simulink model "UGRP_Drone_Modeling4_with_motor_dynamics_v2_with_state_space"  (R2021b)
settings: Solver=FixedStepAuto  StartTime=0.0  StopTime=27  FixedStep=1/600
undefined symbols (not defined in the file or in its folder): sigbuilder_block
libraries: simulink x1, sim3dlib x1, uavsim3dlib x1
settings Model: Creator=user  LastModifiedBy=user
settings SolverCC: MaxConsecutiveMinStep=5  ShapePreserveControl=EnableAll  ZeroCrossAlgorithm=Adaptive
settings DebuggingCC: MaskedZcDiagnostic=none  IgnoredZcDiagnostic=none
settings SFSimCC: SimHardwareAcceleration=native  SimTargetLang=C++

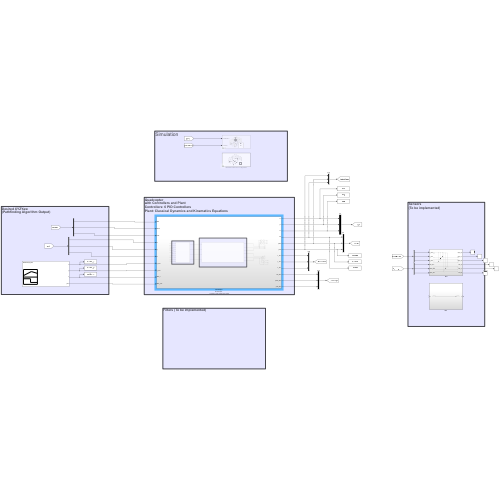
[thumbnail: Simulink's stored preview of the top-level diagram]
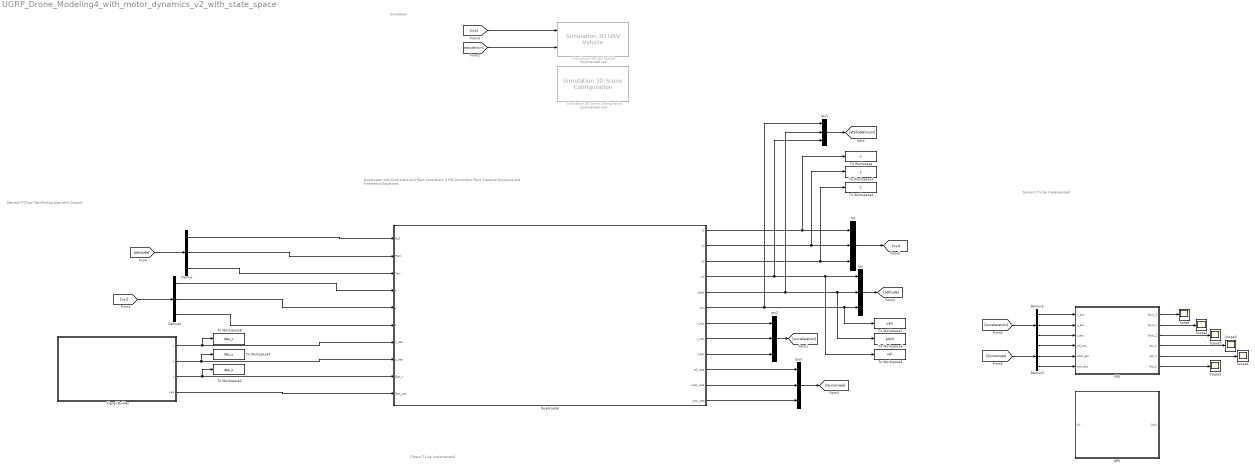
== system UGRP_Drone_Modeling4_with_motor_dynamics_v2_with_state_space ==
  note: Filters (To be implemented)
  note: Sensors
      | (To be implemented)
  note: Desired XYZYaw
      | (Pathfinding Algorithm Output)
  note: Quadcopter
      | with Controllers and Plant
      | Controllers: 6 PID Controllers
      | Plant: Classical Dynamics and Kinematics Equations
  note: Simulation
  Demux{,1..3} (4 alike) : Demux  Outputs=3
  GPS : Subsystem
  IMU : Subsystem
  Quadcopter : Subsystem  Description=Quadcopter including controllers and plant
      settings: AttributesFormatString=|
      | Quadcopter
      | - Controller and Quadcopter Plant
  Scope{,1..5} (6 alike) : Scope
  Signal Builder : Subsystem  Tag=STV Subsys  LoadFcn=sigbuilder_block('load',[10.5 -27.75 821.25 385.5 ]);  StartFcn=sigbuilder_block('start');  StopFcn=sigbuilder_block('stop');  ClipboardFcn=sigbuilder_block('clipboard');  mask(Sigbuilder block){tuvar=[0:10]}
      mask help: Simulink:masks:SigbuilderBlock_MD
      mask init:
      | if ~strcmp(get_param(bdroot(gcbh),'SimulationStatus'),'stopped') tuvar = sigbuilder_block('maskInit'); end
      settings: CopyFcn=sigbuilder_block('copy');  DeleteFcn=sigbuilder_block('delete');  ModelCloseFcn=sigbuilder_block('modelClose');  PreSaveFcn=sigbuilder_block('preSave');  PauseFcn=sigbuilder_block('pause');  ContinueFcn=sigbuilder_block('continue');  NameChangeFcn=sigbuilder_block('namechange');  OpenFcn=sigbuilder_block('open',[9 69.75 821.25 385.5 ]);  CloseFcn=sigbuilder_block('close');
      mask Display: plot(0, 0, 100, 100,[2, 2, 32, 32, 2], [68, 8, 8, 68, 68],[32, 2], [38, 38], [32, 19, 2],[53, 60, 44], [32, 17, 17, 2],[16, 16, 31, 31]);txt = getActiveGroup(gcbh);text(2, 100, txt,'verticalAlignment', 'top');
  Simulation 3D Scene Configuration : sim3dlib/Simulation 3D Scene Configuration  Priority=0  Commented=on  ProjectFormat_internal=Default Scenes  ProjectFormat=Default Scenes  SceneDesc=US city block  ProjectName=C:\Program Files\MATLAB\R2021b\toolbox\shared\sim3d_projects\automotive_project\UE4\WindowsNoEditor\VehicleSimulation.exe  ScenePath=/Game/Maps/USCityBlock  vehTagList={'Scene Origin';'SimulinkVehicle1'}  vehTag=SimulinkVehicle1  OpVisEn=off  Ts=1/60  EnableWindow=on  EnableWeather=off  SunAltitude=40.0  SunAzimuth=90  clouds=10  wind=1  fog=0  rain=0  sensorTag=MainCamera1  sensorId=1  sensorName=MainCamera1  mountLoc=Origin  offsetFlag=off  tmountOffset=[0, 0, 0]  rmountOffset=[0, 0, 0]  HorizontalResolution=1280  VerticalResolution=720  HorizontalFOV=60  mountPoint=[0 0 0]  mountOrientation=[0 0 0]  aMode=4  ID=1
      settings: SourceProductBaseCode=AE,DR,UV,VE
  Simulation 3D UAV Vehicle : uavsim3dlib/Simulation 3D UAV Vehicle  Priority=-1  Commented=on  Mesh=Quadrotor  MeshPath=/MathWorksUAVContent/UAVs/HexaRotorUAV/HexaRotor.HexaRotor  Color=Black  ActorName=SimulinkVehicle1  InitialTranslation=[0 0 0]  InitialRotation=[0 0 0]  SampleTime=-1  ActorType=SimulinkVehicle  ID=1  aMode=4  ActorTag=SimulinkVehicle1
      settings: SourceProductBaseCode=UV
  To Workspace : ToWorkspace  VariableName=x  SaveFormat=Timeseries  SampleTime=-1
  To Workspace2 : ToWorkspace  VariableName=des_z  SaveFormat=Timeseries  SampleTime=-1
  To Workspace3 : ToWorkspace  VariableName=y  SaveFormat=Timeseries  SampleTime=-1
  To Workspace4 : ToWorkspace  VariableName=z  SaveFormat=Timeseries  SampleTime=-1
  To Workspace5 : ToWorkspace  VariableName=roll  SaveFormat=Timeseries  SampleTime=-1
  To Workspace6 : ToWorkspace  VariableName=pitch  SaveFormat=Timeseries  SampleTime=-1
  To Workspace7 : ToWorkspace  VariableName=yaw  SaveFormat=Timeseries  SampleTime=-1
  To Workspace8 : ToWorkspace  VariableName=des_x  SaveFormat=Timeseries  SampleTime=-1
  To Workspace9 : ToWorkspace  VariableName=des_y  SaveFormat=Timeseries  SampleTime=-1
  rpy{,1..3} (4 alike) : Mux  Inputs=3
  xyz : Mux  Inputs=3
  wires:
  Signal Builder/3(z) -> Quadcopter/9(Des_z), To Workspace2/1
  xyz/1 -> [xyz]
  rpy/1 -> [attitude]
  [xyz] -> Demux2/1
  [attitude] -> Demux/1
  Demux2/1 -> Quadcopter/4(x)
  Demux2/2 -> Quadcopter/5(y)
  Demux2/3 -> Quadcopter/6(z)
  Signal Builder/4(yaw) -> Quadcopter/10(Des_yaw)
  [xyz] -> Simulation 3D UAV Vehicle/1
  [attitudeforsim] -> Simulation 3D UAV Vehicle/2
  Signal Builder/1(x) -> Quadcopter/7(x_des), To Workspace8/1
  Signal Builder/2(y) -> Quadcopter/8(y_des), To Workspace9/1
  Quadcopter/1(x1) -> xyz/1, To Workspace/1
  Quadcopter/3(z1) -> To Workspace4/1, xyz/3
  Quadcopter/2(y1) -> To Workspace3/1, xyz/2
  Demux/1 -> Quadcopter/1(Roll)
  Demux/2 -> Quadcopter/2(Pitch)
  Demux/3 -> Quadcopter/3(Yaw)
  rpy1/1 -> [attitudeforsim]
  Quadcopter/4(roll) -> rpy1/3, To Workspace5/1, rpy/1
  Quadcopter/5(pitch) -> rpy1/2, To Workspace6/1, rpy/2
  Quadcopter/6(yaw) -> rpy1/1, To Workspace7/1, rpy/3
  Quadcopter/7(x_acc) -> rpy2/1
  Quadcopter/8(y_acc) -> rpy2/2
  Quadcopter/9(z_acc) -> rpy2/3
  Quadcopter/10(roll_rate) -> rpy3/1
  Quadcopter/11(pitch_rate) -> rpy3/2
  Quadcopter/12(yaw_rate) -> rpy3/3
  rpy2/1 -> [Acceleration]
  rpy3/1 -> [Gyroscope]
  [Acceleration] -> Demux1/1
  [Gyroscope] -> Demux3/1
  Demux1/1 -> IMU/1(x_acc)
  Demux1/2 -> IMU/2(y_acc)
  Demux1/3 -> IMU/3(z_acc)
  Demux3/1 -> IMU/4(roll_acc)
  Demux3/2 -> IMU/5(pitch_acc)
  Demux3/3 -> IMU/6(yaw_acc)
  IMU/1(Gyro_X) -> Scope/1
  IMU/2(Gyro_Y) -> Scope1/1
  IMU/3(Gyro_Z) -> Scope2/1
  IMU/4(Acc_X) -> Scope3/1
  IMU/5(Acc_Y) -> Scope4/1
  IMU/6(Acc_Z) -> Scope5/1

== system UGRP_Drone_Modeling4_with_motor_dynamics_v2_with_state_space/GPS ==
  In1 : Inport
  Out1 : Outport
  wires:
  In1/1 -> Out1/1

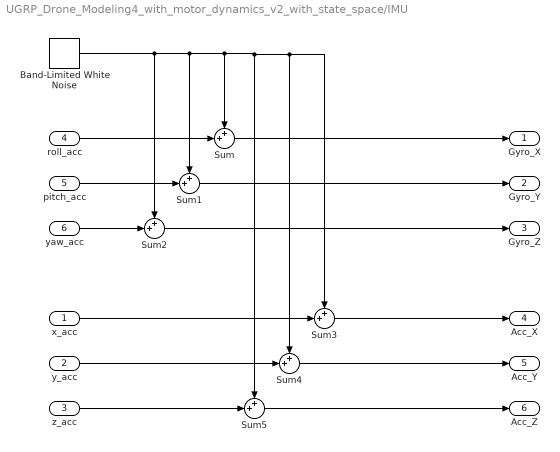
== system UGRP_Drone_Modeling4_with_motor_dynamics_v2_with_state_space/IMU ==
  x_acc : Inport
  y_acc : Inport  Port=2
  z_acc : Inport  Port=3
  roll_acc : Inport  Port=4
  pitch_acc : Inport  Port=5
  yaw_acc : Inport  Port=6
  Band-Limited White Noise : simulink/Sources/Band-Limited White Noise  Cov=[0.5]  Ts=0.1  seed=[23341]
  Sum{,1..5} (6 alike) : Sum  Inputs=++|
  Gyro_X : Outport
  Gyro_Y : Outport  Port=2
  Gyro_Z : Outport  Port=3
  Acc_X : Outport  Port=4
  Acc_Y : Outport  Port=5
  Acc_Z : Outport  Port=6
  wires:
  yaw_acc/1 -> Sum2/2
  pitch_acc/1 -> Sum1/2
  roll_acc/1 -> Sum/2
  Band-Limited White Noise/1 -> Sum3/1, Sum4/1, Sum5/1, Sum/1, Sum1/1, Sum2/1
  x_acc/1 -> Sum3/2
  y_acc/1 -> Sum4/2
  z_acc/1 -> Sum5/2
  Sum/1 -> Gyro_X/1
  Sum1/1 -> Gyro_Y/1
  Sum2/1 -> Gyro_Z/1
  Sum3/1 -> Acc_X/1
  Sum4/1 -> Acc_Y/1
  Sum5/1 -> Acc_Z/1

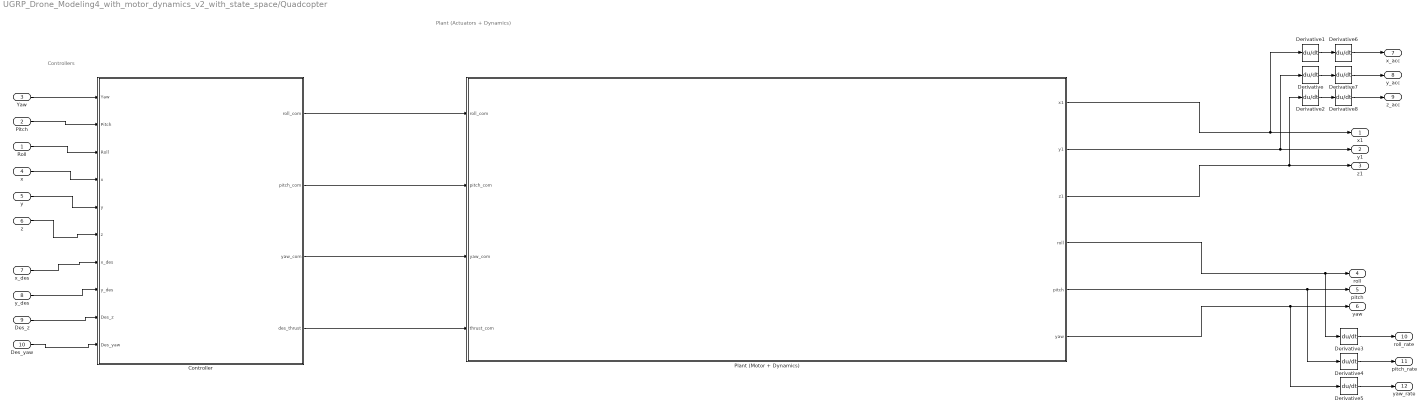
== system UGRP_Drone_Modeling4_with_motor_dynamics_v2_with_state_space/Quadcopter ==
  note: Plant (Actuators + Dynamics)
  note: Controllers
  Roll : Inport
  Pitch : Inport  Port=2
  Yaw : Inport  Port=3
  x : Inport  Port=4
  y : Inport  Port=5
  z : Inport  Port=6
  x_des : Inport  Port=7
  y_des : Inport  Port=8
  Des_z : Inport  Port=9
  Des_yaw : Inport  Port=10
  Controller : Subsystem
  Derivative{,1..8} (9 alike) : Derivative
  Plant (Motor + Dynamics) : Subsystem
  x1 : Outport
  y1 : Outport  Port=2
  z1 : Outport  Port=3
  roll : Outport  Port=4
  pitch : Outport  Port=5
  yaw : Outport  Port=6
  x_acc : Outport  Port=7
  y_acc : Outport  Port=8
  z_acc : Outport  Port=9
  roll_rate : Outport  Port=10
  pitch_rate : Outport  Port=11
  yaw_rate : Outport  Port=12
  wires:
  x_des/1 -> Controller/7(x_des)
  Controller/1(roll_com) -> Plant (Motor + Dynamics)/1(roll_com)
  Controller/2(pitch_com) -> Plant (Motor + Dynamics)/2(pitch_com)
  Des_yaw/1 -> Controller/10(Des_yaw)
  Controller/4(des_thrust) -> Plant (Motor + Dynamics)/4(thrust_com)
  Controller/3(yaw_com) -> Plant (Motor + Dynamics)/3(yaw_com)
  y/1 -> Controller/5(y)
  Des_z/1 -> Controller/9(Des_z)
  x/1 -> Controller/4(x)
  Roll/1 -> Controller/3(Roll)
  y_des/1 -> Controller/8(y_des)
  Yaw/1 -> Controller/1(Yaw)
  z/1 -> Controller/6(z)
  Pitch/1 -> Controller/2(Pitch)
  Plant (Motor + Dynamics)/2(y1) -> Derivative/1, y1/1
  Plant (Motor + Dynamics)/1(x1) -> Derivative1/1, x1/1
  Plant (Motor + Dynamics)/6(yaw) -> Derivative5/1, yaw/1
  Plant (Motor + Dynamics)/5(pitch) -> Derivative4/1, pitch/1
  Plant (Motor + Dynamics)/3(z1) -> Derivative2/1, z1/1
  Plant (Motor + Dynamics)/4(roll) -> Derivative3/1, roll/1
  Derivative1/1 -> Derivative6/1
  Derivative/1 -> Derivative7/1
  Derivative2/1 -> Derivative8/1
  Derivative3/1 -> roll_rate/1
  Derivative4/1 -> pitch_rate/1
  Derivative5/1 -> yaw_rate/1
  Derivative6/1 -> x_acc/1
  Derivative7/1 -> y_acc/1
  Derivative8/1 -> z_acc/1

== system UGRP_Drone_Modeling4_with_motor_dynamics_v2_with_state_space/Signal Builder ==
  Demux : Demux  Tag=STV Demux
      settings: DisplayOption=none
  FromWs : FromWorkspace  Tag=STV FromWs  VariableName=tuvar
      SigBuilderData=|
      | common.afterFinalStr = 'Extrapolate'
      | common.sampleTime = 0
      | dataSet.timeRange = [0 25]
      | dataSet.name = 'Desired xyzyaw'
      | sbobj.Groups.Name = 'Desired xyzyaw'
      | sbobj.Groups.Signals(1).Name = 'x'
      | sbobj.Groups.Signals(1).XData = [0 10 10 15 25]
      | sbobj.Groups.Signals(1).YData = [0 0 2 2 2]
      | sbobj.Groups.Signals(2).Name = 'y'
      | sbobj.Groups.Signals(2).XData = [0 3.99 15 18 18 25]
      | sbobj.Groups.Signals(2).YData = [0 0 0 0 2 2]
      | sbobj.Groups.Signals(3).Name = 'z'
      | sbobj.Groups.Signals(3).XData = [0 25]
      | sbobj.Groups.Signals(3).YData = [3 3]
      | sbobj.Groups.Signals(4).Name = 'yaw'
      | sbobj.Groups.Signals(4).XData = [0 5 8 25]
      | sbobj.Groups.Signals(4).YData = [0 0 0 0]
      | sbobj.Groups.TimeRange = [0 25]
  x : Outport  Tag=STV Outport
  y : Outport  Tag=STV Outport  Port=2
  z : Outport  Tag=STV Outport  Port=3
  yaw : Outport  Tag=STV Outport  Port=4
  wires:
  FromWs/1 -> Demux/1
  Demux/1 -> x/1
  Demux/2 -> y/1
  Demux/3 -> z/1
  Demux/4 -> yaw/1

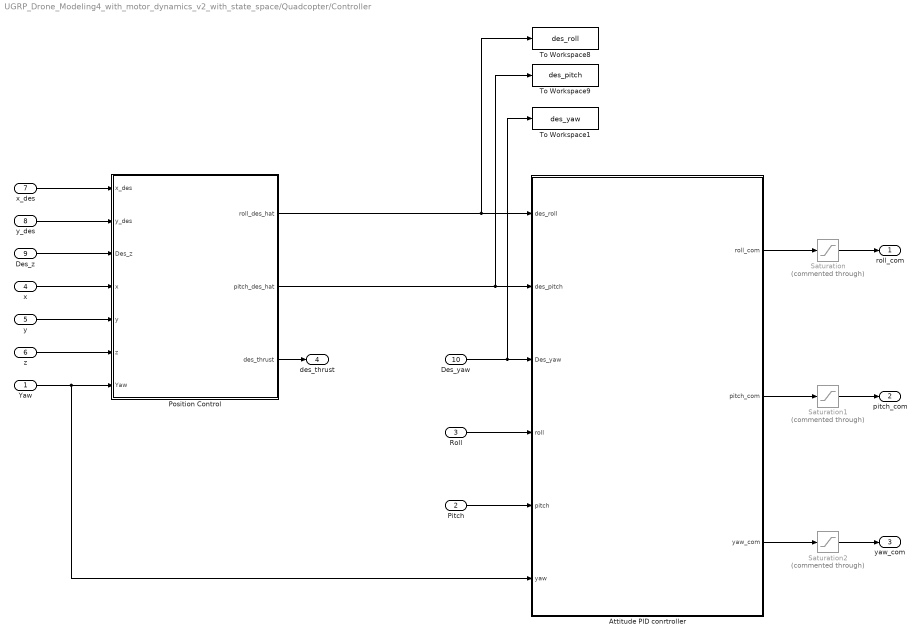
== system UGRP_Drone_Modeling4_with_motor_dynamics_v2_with_state_space/Quadcopter/Controller ==
  Yaw : Inport
  Pitch : Inport  Port=2
  Roll : Inport  Port=3
  x : Inport  Port=4
  y : Inport  Port=5
  z : Inport  Port=6
  x_des : Inport  Port=7
  y_des : Inport  Port=8
  Des_z : Inport  Port=9
  Des_yaw : Inport  Port=10
  Attitude PID conrtroller : Subsystem
  Position Control : Subsystem
  Saturation : Saturate  Commented=through  UpperLimit=4  LowerLimit=-4
  Saturation1 : Saturate  Commented=through  UpperLimit=1  LowerLimit=-1
  Saturation2 : Saturate  Commented=through  UpperLimit=1  LowerLimit=-1
  To Workspace1 : ToWorkspace  VariableName=des_yaw  SaveFormat=Timeseries  SampleTime=-1
  To Workspace8 : ToWorkspace  VariableName=des_roll  SaveFormat=Timeseries  SampleTime=-1
  To Workspace9 : ToWorkspace  VariableName=des_pitch  SaveFormat=Timeseries  SampleTime=-1
  roll_com : Outport
  pitch_com : Outport  Port=2
  yaw_com : Outport  Port=3
  des_thrust : Outport  Port=4
  wires:
  Attitude PID conrtroller/2(pitch_com) -> Saturation1/1
  Position Control/3(des_thrust) -> des_thrust/1
  y/1 -> Position Control/5(y)
  Attitude PID conrtroller/3(yaw_com) -> Saturation2/1
  Attitude PID conrtroller/1(roll_com) -> Saturation/1
  Des_yaw/1 -> Attitude PID conrtroller/3(Des_yaw), To Workspace1/1
  x_des/1 -> Position Control/1(x_des)
  z/1 -> Position Control/6(z)
  Des_z/1 -> Position Control/3(Des_z)
  y_des/1 -> Position Control/2(y_des)
  Yaw/1 -> Attitude PID conrtroller/6(yaw), Position Control/7(Yaw)
  x/1 -> Position Control/4(x)
  Position Control/2(pitch_des_hat) -> Attitude PID conrtroller/2(des_pitch), To Workspace9/1
  Position Control/1(roll_des_hat) -> Attitude PID conrtroller/1(des_roll), To Workspace8/1
  Roll/1 -> Attitude PID conrtroller/4(roll)
  Pitch/1 -> Attitude PID conrtroller/5(pitch)
  Saturation/1 -> roll_com/1
  Saturation1/1 -> pitch_com/1
  Saturation2/1 -> yaw_com/1

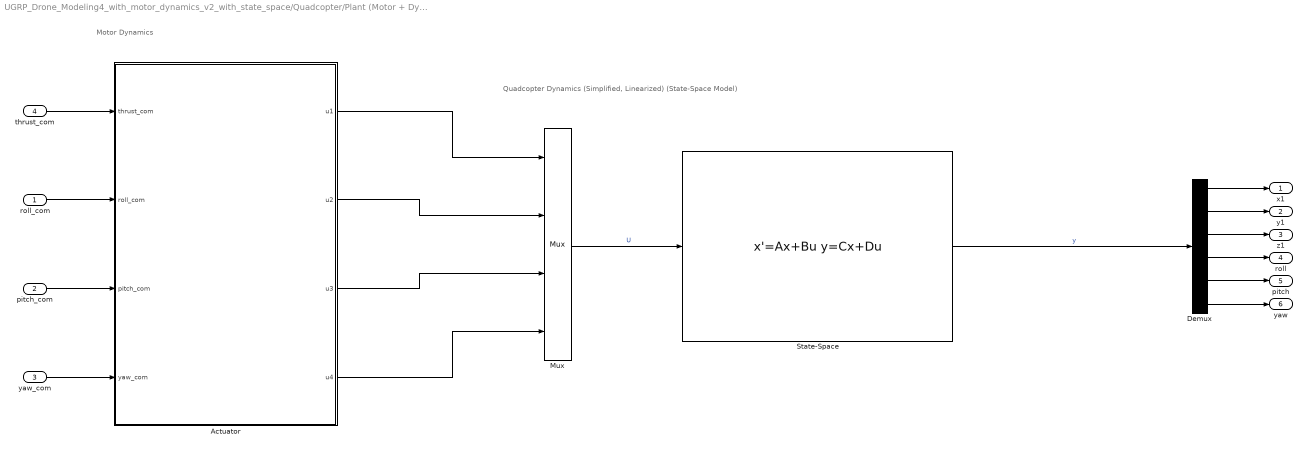
== system UGRP_Drone_Modeling4_with_motor_dynamics_v2_with_state_space/Quadcopter/Plant (Motor + Dynamics) ==
  note: Motor Dynamics
  note: Quadcopter Dynamics  (Simplified, Linearized)
      | (State-Space Model)
  roll_com : Inport
  pitch_com : Inport  Port=2
  yaw_com : Inport  Port=3
  thrust_com : Inport  Port=4
  Actuator : Subsystem
  Demux : Demux  Outputs=6
  Mux : Mux
  State-Space : StateSpace  A=|  B=|  C=|  D=|  InitialCondition=[0 0 0 0 0 0 0 0 0 0 0 0]  ContinuousStateAttributes='state'
      A=|
      | [0 0 0 0 0 0 1 0 0 0 0 0 ; 
      |      0 0 0 0 0 0 0 1 0 0 0 0 ;
      |      0 0 0 0 0 0 0 0 1 0 0 0 ;
      |      0 0 0 0 0 0 0 0 0 1 0 0 ;
      |      0 0 0 0 0 0 0 0 0 0 1 0 ;
      |      0 0 0 0 0 0 0 0 0 0 0 1 ;
      |      0 0 0 0 9.80 0 0 0 0 0 0 0 ;
      |      0 0 0 -9.80 0 0 0 0 0 0 0 0 ;
      |      0 0 0 0 0 0 0 0 0 0 0 0 ;
      |      0 0 0 0 0 0 0 0 0 0 0 0 ;
      |      0 0 0 0 0 0 0 0 0 0 0 0 ;
      |      0 0 0 0 0 0 0 0 0 0 0 0]
      B=|
      | [0 0 0 0;
      |      0 0 0 0;
      |      0 0 0 0;
      |      0 0 0 0;
      |      0 0 0 0;
      |      0 0 0 0;
      |      0 0 0 0;
      |      0 0 0 0;
      |      (1/1.568) 0 0 0;
      |      0 (1/0.0090) 0 0;
      |      0 0 (1/0.0090) 0;
      |      0 0 0 (1/0.017)]
      C=|
      | [1 0 0 0 0 0 0 0 0 0 0 0;
      |      0 1 0 0 0 0 0 0 0 0 0 0;
      |      0 0 1 0 0 0 0 0 0 0 0 0;
      |      0 0 0 1 0 0 0 0 0 0 0 0;
      |      0 0 0 0 1 0 0 0 0 0 0 0;
      |      0 0 0 0 0 1 0 0 0 0 0 0]
      D=|
      | [0 0 0 0 ; 
      |      0 0 0 0 ;
      |      0 0 0 0 ;
      |      0 0 0 0 ;
      |      0 0 0 0 ;
      |      0 0 0 0 ]
  x1 : Outport
  y1 : Outport  Port=2
  z1 : Outport  Port=3
  roll : Outport  Port=4
  pitch : Outport  Port=5
  yaw : Outport  Port=6
  wires:
  Mux/1 -> State-Space/1  "U"
  roll_com/1 -> Actuator/2(roll_com)
  pitch_com/1 -> Actuator/3(pitch_com)
  yaw_com/1 -> Actuator/4(yaw_com)
  Actuator/2(u2) -> Mux/2
  Actuator/3(u3) -> Mux/3
  Actuator/4(u4) -> Mux/4
  State-Space/1 -> Demux/1  "y"
  Demux/5 -> pitch/1
  Demux/1 -> x1/1
  Demux/3 -> z1/1
  Demux/2 -> y1/1
  Demux/6 -> yaw/1
  Demux/4 -> roll/1
  thrust_com/1 -> Actuator/1(thrust_com)
  Actuator/1(u1) -> Mux/1

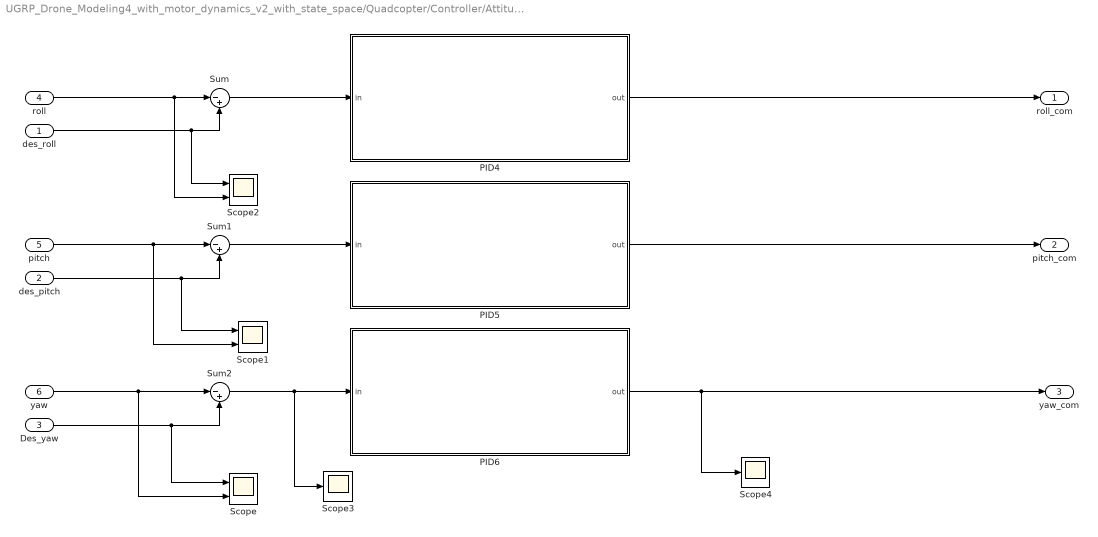
== system UGRP_Drone_Modeling4_with_motor_dynamics_v2_with_state_space/Quadcopter/Controller/Attitude PID conrtroller ==
  des_roll : Inport
  des_pitch : Inport  Port=2
  Des_yaw : Inport  Port=3
  roll : Inport  Port=4
  pitch : Inport  Port=5
  yaw : Inport  Port=6
  PID4 : Subsystem
  PID5 : Subsystem
  PID6 : Subsystem
  Scope : Scope  NumInputPorts=2
  Scope1 : Scope  NumInputPorts=2
  Scope2 : Scope  NumInputPorts=2
  Scope3 : Scope
  Scope4 : Scope
  Sum : Sum  Inputs=|-+
  Sum1 : Sum  Inputs=|-+
  Sum2 : Sum  Inputs=|-+
  roll_com : Outport
  pitch_com : Outport  Port=2
  yaw_com : Outport  Port=3
  wires:
  des_roll/1 -> Scope2/1, Sum/2
  Des_yaw/1 -> Scope/1, Sum2/2
  yaw/1 -> Scope/2, Sum2/1
  Sum/1 -> PID4/1(in)
  Sum2/1 -> Scope3/1, PID6/1(in)
  Sum1/1 -> PID5/1(in)
  pitch/1 -> Scope1/2, Sum1/1
  des_pitch/1 -> Scope1/1, Sum1/2
  roll/1 -> Scope2/2, Sum/1
  PID4/1(out) -> roll_com/1
  PID5/1(out) -> pitch_com/1
  PID6/1(out) -> Scope4/1, yaw_com/1

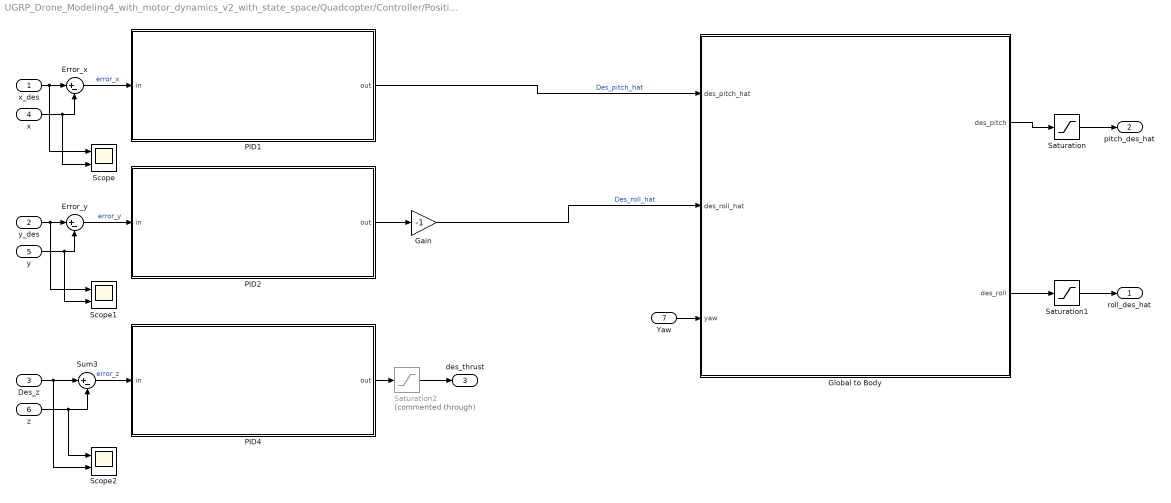
== system UGRP_Drone_Modeling4_with_motor_dynamics_v2_with_state_space/Quadcopter/Controller/Position Control ==
  x_des : Inport
  y_des : Inport  Port=2
  Des_z : Inport  Port=3
  x : Inport  Port=4
  y : Inport  Port=5
  z : Inport  Port=6
  Yaw : Inport  Port=7
  Error_x : Sum  Inputs=|+-
  Error_y : Sum  Inputs=|+-
  Gain : Gain  Gain=-1
  Global to Body : Subsystem
  PID1 : Subsystem
  PID2 : Subsystem
  PID4 : Subsystem
  Saturation : Saturate  UpperLimit=10*pi/180  LowerLimit=-10*pi/180
  Saturation1 : Saturate  UpperLimit=10*pi/180  LowerLimit=-10*pi/180
  Saturation2 : Saturate  Commented=through  UpperLimit=17  LowerLimit=0
  Scope : Scope  NumInputPorts=2
  Scope1 : Scope  NumInputPorts=2
  Scope2 : Scope  NumInputPorts=2
  Sum3 : Sum  Inputs=|+-
  roll_des_hat : Outport
  pitch_des_hat : Outport  Port=2
  des_thrust : Outport  Port=3
  wires:
  x_des/1 -> Scope/1, Error_x/1
  x/1 -> Scope/2, Error_x/2
  y_des/1 -> Scope1/1, Error_y/1
  y/1 -> Scope1/2, Error_y/2
  Des_z/1 -> Scope2/2, Sum3/1
  Yaw/1 -> Global to Body/3(yaw)
  Error_y/1 -> PID2/1(in)  "error_y"
  Error_x/1 -> PID1/1(in)  "error_x"
  Global to Body/2(des_roll) -> Saturation1/1
  z/1 -> Scope2/1, Sum3/2
  Global to Body/1(des_pitch) -> Saturation/1
  PID1/1(out) -> Global to Body/1(des_pitch_hat)  "Des_pitch_hat"
  PID2/1(out) -> Gain/1
  Gain/1 -> Global to Body/2(des_roll_hat)  "Des_roll_hat"
  Saturation1/1 -> roll_des_hat/1
  Saturation/1 -> pitch_des_hat/1
  Sum3/1 -> PID4/1(in)  "error_z"
  PID4/1(out) -> Saturation2/1
  Saturation2/1 -> des_thrust/1

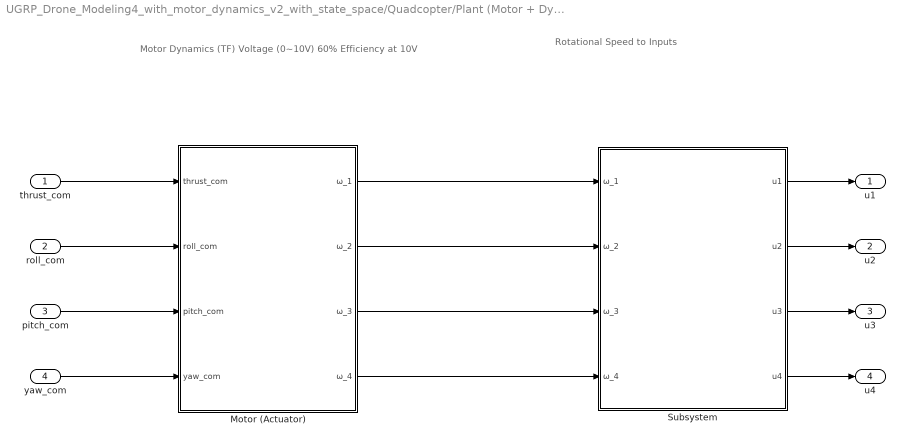
== system UGRP_Drone_Modeling4_with_motor_dynamics_v2_with_state_space/Quadcopter/Plant (Motor + Dynamics)/Actuator ==
  note: Rotational Speed
      | to Inputs
  note: Motor Dynamics (TF)
      | Voltage (0~10V)
      | 60% Efficiency at 10V
  thrust_com : Inport
  roll_com : Inport  Port=2
  pitch_com : Inport  Port=3
  yaw_com : Inport  Port=4
  Motor (Actuator) : Subsystem
  Subsystem : Subsystem
  u1 : Outport
  u2 : Outport  Port=2
  u3 : Outport  Port=3
  u4 : Outport  Port=4
  wires:
  thrust_com/1 -> Motor (Actuator)/1(thrust_com)
  Motor (Actuator)/4(ω_4) -> Subsystem/4(ω_4)
  Motor (Actuator)/2(ω_2) -> Subsystem/2(ω_2)
  yaw_com/1 -> Motor (Actuator)/4(yaw_com)
  Motor (Actuator)/3(ω_3) -> Subsystem/3(ω_3)
  Motor (Actuator)/1(ω_1) -> Subsystem/1(ω_1)
  pitch_com/1 -> Motor (Actuator)/3(pitch_com)
  Subsystem/4(u4) -> u4/1
  roll_com/1 -> Motor (Actuator)/2(roll_com)
  Subsystem/3(u3) -> u3/1
  Subsystem/2(u2) -> u2/1
  Subsystem/1(u1) -> u1/1

== system UGRP_Drone_Modeling4_with_motor_dynamics_v2_with_state_space/Quadcopter/Controller/Attitude PID conrtroller/PID4 ==
  in : Inport
  Add1 : Sum  Inputs=+++
  Derivative : Derivative
  Gain : Gain  Gain=2.5
  Gain1 : Gain  Gain=0
  Gain2 : Gain  Gain=0.345
  Integrator Limited : Integrator  LimitOutput=on  UpperSaturationLimit=10  LowerSaturationLimit=-10
  out : Outport
  wires:
  Integrator Limited/1 -> Gain1/1
  Gain/1 -> Add1/1
  Gain1/1 -> Add1/2
  Derivative/1 -> Gain2/1
  Gain2/1 -> Add1/3
  Add1/1 -> out/1
  in/1 -> Derivative/1, Gain/1, Integrator Limited/1

== system UGRP_Drone_Modeling4_with_motor_dynamics_v2_with_state_space/Quadcopter/Controller/Attitude PID conrtroller/PID5 ==
  in : Inport
  Add1 : Sum  Inputs=+++
  Derivative : Derivative
  Gain : Gain  Gain=2.5
  Gain1 : Gain  Gain=0
  Gain2 : Gain  Gain=0.345
  Integrator Limited : Integrator  LimitOutput=on  UpperSaturationLimit=10  LowerSaturationLimit=-10
  out : Outport
  wires:
  Integrator Limited/1 -> Gain1/1
  Gain/1 -> Add1/1
  Gain1/1 -> Add1/2
  Derivative/1 -> Gain2/1
  Gain2/1 -> Add1/3
  Add1/1 -> out/1
  in/1 -> Derivative/1, Gain/1, Integrator Limited/1

== system UGRP_Drone_Modeling4_with_motor_dynamics_v2_with_state_space/Quadcopter/Controller/Attitude PID conrtroller/PID6 ==
  in : Inport
  Add1 : Sum  Inputs=+++
  Derivative : Derivative
  Gain : Gain
  Gain1 : Gain  Gain=0
  Gain2 : Gain  Gain=0.06
  Integrator Limited : Integrator  LimitOutput=on  UpperSaturationLimit=10  LowerSaturationLimit=-10
  out : Outport
  wires:
  Integrator Limited/1 -> Gain1/1
  Gain/1 -> Add1/1
  in/1 -> Derivative/1, Gain/1, Integrator Limited/1
  Gain1/1 -> Add1/2
  Derivative/1 -> Gain2/1
  Gain2/1 -> Add1/3
  Add1/1 -> out/1

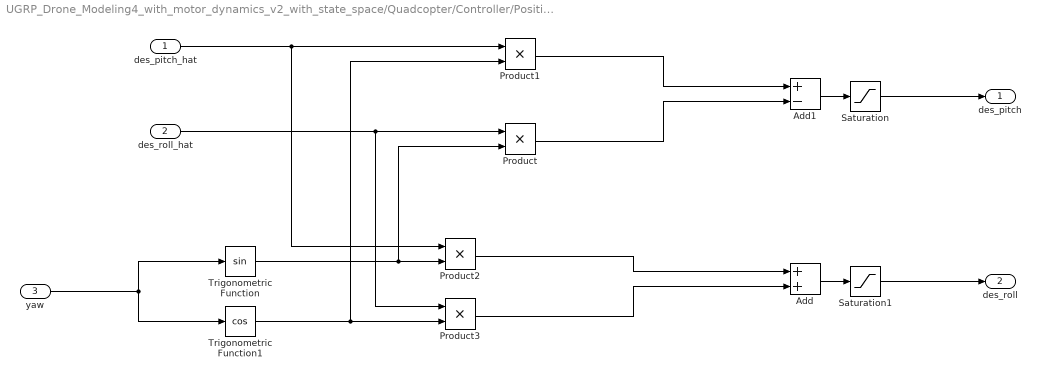
== system UGRP_Drone_Modeling4_with_motor_dynamics_v2_with_state_space/Quadcopter/Controller/Position Control/Global to Body ==
  des_pitch_hat : Inport
  des_roll_hat : Inport  Port=2
  yaw : Inport  Port=3
  Add : Sum
  Add1 : Sum  Inputs=+-
  Product{,1..3} (4 alike) : Product
  Saturation : Saturate  UpperLimit=10*pi/180  LowerLimit=-10*pi/180
  Saturation1 : Saturate  UpperLimit=10*pi/180  LowerLimit=-10*pi/180
  Trigonometric Function : Trigonometry
  Trigonometric Function1 : Trigonometry  Operator=cos
  des_pitch : Outport
  des_roll : Outport  Port=2
  wires:
  yaw/1 -> Trigonometric Function/1, Trigonometric Function1/1
  Add/1 -> Saturation1/1
  Add1/1 -> Saturation/1
  Saturation1/1 -> des_roll/1
  des_pitch_hat/1 -> Product2/1, Product1/1
  Product1/1 -> Add1/1
  Trigonometric Function1/1 -> Product3/2, Product1/2
  des_roll_hat/1 -> Product3/1, Product/1
  Trigonometric Function/1 -> Product2/2, Product/2
  Product/1 -> Add1/2
  Product2/1 -> Add/1
  Product3/1 -> Add/2
  Saturation/1 -> des_pitch/1

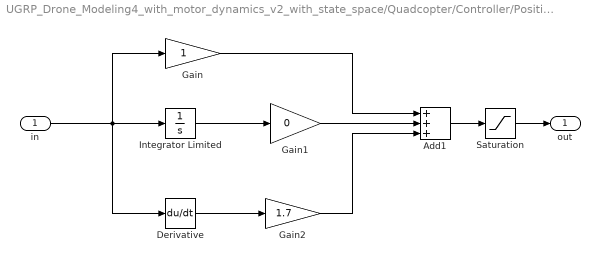
== system UGRP_Drone_Modeling4_with_motor_dynamics_v2_with_state_space/Quadcopter/Controller/Position Control/PID1 ==
  in : Inport
  Add1 : Sum  Inputs=+++
  Derivative : Derivative
  Gain : Gain
  Gain1 : Gain  Gain=0
  Gain2 : Gain  Gain=1.7
  Integrator Limited : Integrator  LimitOutput=on  UpperSaturationLimit=20  LowerSaturationLimit=-20
  Saturation : Saturate  UpperLimit=10*pi/180  LowerLimit=-10*pi/180
  out : Outport
  wires:
  Integrator Limited/1 -> Gain1/1
  in/1 -> Derivative/1, Gain/1, Integrator Limited/1
  Gain/1 -> Add1/1
  Gain1/1 -> Add1/2
  Derivative/1 -> Gain2/1
  Gain2/1 -> Add1/3
  Add1/1 -> Saturation/1
  Saturation/1 -> out/1

== system UGRP_Drone_Modeling4_with_motor_dynamics_v2_with_state_space/Quadcopter/Controller/Position Control/PID2 ==
  in : Inport
  Add1 : Sum  Inputs=+++
  Derivative : Derivative
  Gain : Gain
  Gain1 : Gain  Gain=0
  Gain2 : Gain  Gain=1.7
  Integrator Limited : Integrator  LimitOutput=on  UpperSaturationLimit=10  LowerSaturationLimit=-10
  Saturation : Saturate  UpperLimit=10*pi/180  LowerLimit=-10*pi/180
  out : Outport
  wires:
  Integrator Limited/1 -> Gain1/1
  in/1 -> Derivative/1, Gain/1, Integrator Limited/1
  Gain/1 -> Add1/1
  Gain1/1 -> Add1/2
  Derivative/1 -> Gain2/1
  Gain2/1 -> Add1/3
  Add1/1 -> Saturation/1
  Saturation/1 -> out/1

== system UGRP_Drone_Modeling4_with_motor_dynamics_v2_with_state_space/Quadcopter/Controller/Position Control/PID4 ==
  in : Inport
  Add1 : Sum  Inputs=+++
  Derivative : Derivative
  Gain : Gain  Gain=4.5
  Gain1 : Gain  Gain=0
  Gain2 : Gain  Gain=1.7
  Integrator Limited : Integrator  LimitOutput=on  UpperSaturationLimit=100  LowerSaturationLimit=-100
  out : Outport
  wires:
  Integrator Limited/1 -> Gain1/1
  Gain/1 -> Add1/1
  in/1 -> Derivative/1, Gain/1, Integrator Limited/1
  Gain1/1 -> Add1/2
  Gain2/1 -> Add1/3
  Add1/1 -> out/1
  Derivative/1 -> Gain2/1

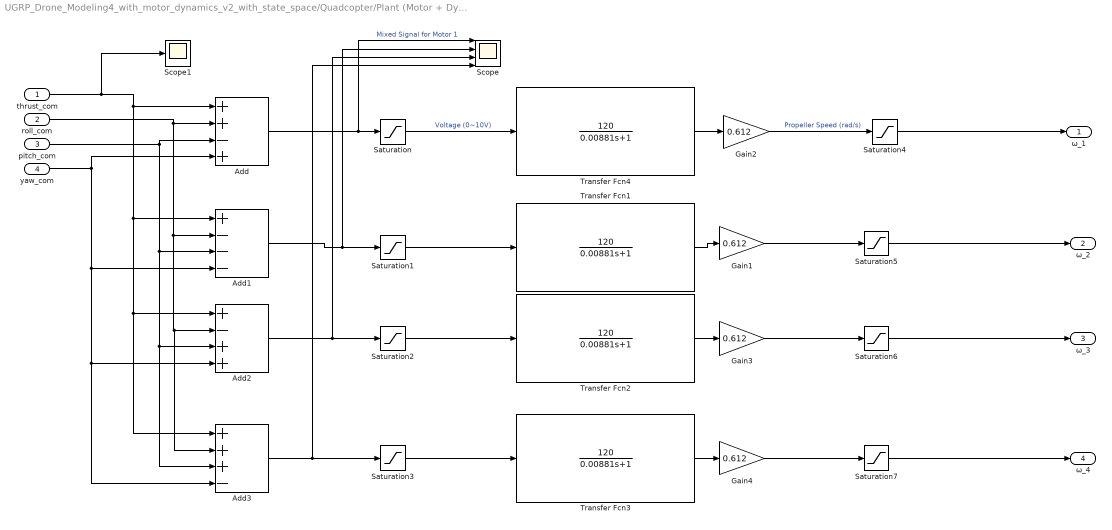
== system UGRP_Drone_Modeling4_with_motor_dynamics_v2_with_state_space/Quadcopter/Plant (Motor + Dynamics)/Actuator/Motor (Actuator) ==
  thrust_com : Inport
  roll_com : Inport  Port=2
  pitch_com : Inport  Port=3
  yaw_com : Inport  Port=4
  Add : Sum  Inputs=++-+
  Add1 : Sum  Inputs=+---
  Add2 : Sum  Inputs=+-++
  Add3 : Sum  Inputs=+++-
  Gain{1..4} (4 alike) : Gain  Gain=0.612
  Saturation{,1..3} (4 alike) : Saturate  UpperLimit=10  LowerLimit=0
  Saturation{4..7} (4 alike) : Saturate  UpperLimit=1040  LowerLimit=0
  Scope : Scope  NumInputPorts=4
  Scope1 : Scope
  Transfer Fcn{1..4} (4 alike) : TransferFcn  Numerator=[120]  Denominator=[0.00881 1]
  ω_1 : Outport
  ω_2 : Outport  Port=2
  ω_3 : Outport  Port=3
  ω_4 : Outport  Port=4
  wires:
  Add/1 -> Scope/1, Saturation/1  "Mixed Signal for Motor 1"
  Add1/1 -> Scope/2, Saturation1/1
  Add2/1 -> Scope/3, Saturation2/1
  Add3/1 -> Scope/4, Saturation3/1
  Saturation/1 -> Transfer Fcn4/1  "Voltage (0~10V)"
  Saturation2/1 -> Transfer Fcn2/1
  Saturation1/1 -> Transfer Fcn1/1
  Saturation3/1 -> Transfer Fcn3/1
  Saturation4/1 -> ω_1/1
  Saturation5/1 -> ω_2/1
  Saturation6/1 -> ω_3/1
  Saturation7/1 -> ω_4/1
  Transfer Fcn4/1 -> Gain2/1
  Gain2/1 -> Saturation4/1  "Propeller Speed (rad/s)"
  Transfer Fcn1/1 -> Gain1/1
  Gain1/1 -> Saturation5/1
  Transfer Fcn2/1 -> Gain3/1
  Gain3/1 -> Saturation6/1
  Transfer Fcn3/1 -> Gain4/1
  Gain4/1 -> Saturation7/1
  thrust_com/1 -> Scope1/1, Add/1, Add3/1, Add2/1, Add1/1
  roll_com/1 -> Add3/2, Add2/2, Add1/2, Add/2
  pitch_com/1 -> Add/3, Add3/3, Add2/3, Add1/3
  yaw_com/1 -> Add3/4, Add2/4, Add1/4, Add/4

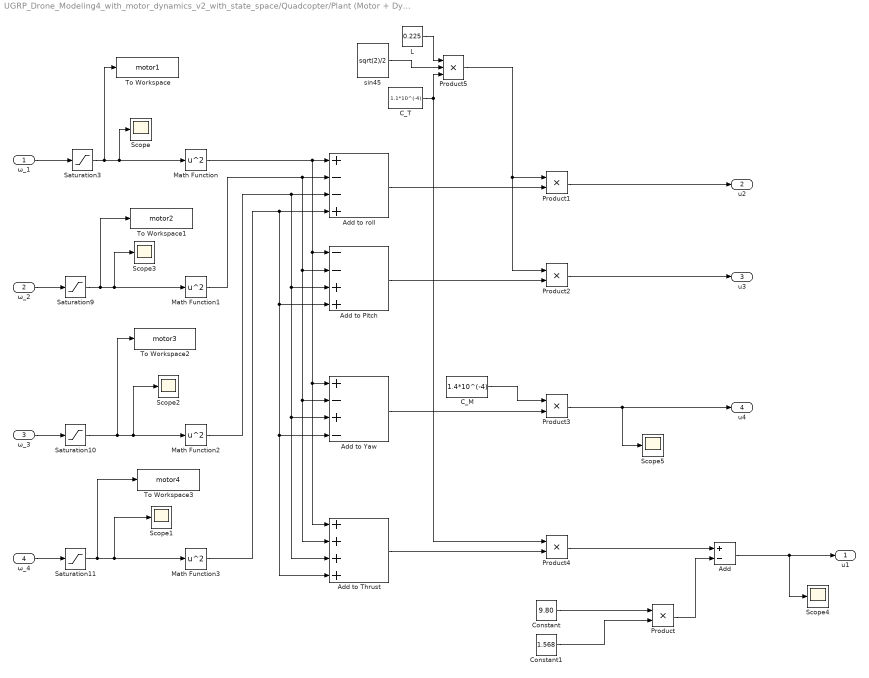
== system UGRP_Drone_Modeling4_with_motor_dynamics_v2_with_state_space/Quadcopter/Plant (Motor + Dynamics)/Actuator/Subsystem ==
  ω_1 : Inport
  ω_2 : Inport  Port=2
  ω_3 : Inport  Port=3
  ω_4 : Inport  Port=4
  Add : Sum  Inputs=+-
  Add to Pitch : Sum  Inputs=--++  RndMeth=Round
  Add to Thrust : Sum  Inputs=++++  RndMeth=Round
  Add to Yaw : Sum  Inputs=+-+-  RndMeth=Round
  Add to roll : Sum  Inputs=+--+
  C_M : Constant  Value=1.4*10^(-4)
  C_T : Constant  Value=1.1*10^(-4)
  Constant : Constant  Value=9.80
  Constant1 : Constant  Value=1.568
  L : Constant  Value=0.225
  Math Function : Math  Operator=square  RndMeth=Round  SaturateOnIntegerOverflow=on
  Math Function1 : Math  Operator=square  SaturateOnIntegerOverflow=on
  Math Function2 : Math  Operator=square  SaturateOnIntegerOverflow=on
  Math Function3 : Math  Operator=square  SaturateOnIntegerOverflow=on
  Product{,1..4} (5 alike) : Product
  Product5 : Product  Inputs=3
  Saturation{3,9..11} (4 alike) : Saturate  UpperLimit=1000  LowerLimit=0
  Scope{,1..5} (6 alike) : Scope
  To Workspace : ToWorkspace  VariableName=motor1  SaveFormat=Timeseries  SampleTime=-1
  To Workspace1 : ToWorkspace  VariableName=motor2  SaveFormat=Timeseries  SampleTime=-1
  To Workspace2 : ToWorkspace  VariableName=motor3  SaveFormat=Timeseries  SampleTime=-1
  To Workspace3 : ToWorkspace  VariableName=motor4  SaveFormat=Timeseries  SampleTime=-1
  sin45 : Constant  Value=sqrt(2)/2
  u1 : Outport
  u2 : Outport  Port=2
  u3 : Outport  Port=3
  u4 : Outport  Port=4
  wires:
  Saturation11/1 -> To Workspace3/1, Scope1/1, Math Function3/1
  Add to roll/1 -> Product1/2
  ω_1/1 -> Saturation3/1
  C_M/1 -> Product3/1
  Add to Yaw/1 -> Product3/2
  Math Function3/1 -> Add to Thrust/4, Add to Yaw/4, Add to Pitch/4, Add to roll/4
  Product5/1 -> Product2/1, Product1/1
  Math Function2/1 -> Add to Thrust/3, Add to Yaw/3, Add to Pitch/3, Add to roll/3
  ω_3/1 -> Saturation10/1
  L/1 -> Product5/1
  sin45/1 -> Product5/2
  Saturation9/1 -> To Workspace1/1, Scope3/1, Math Function1/1
  Add to Thrust/1 -> Product4/2
  Saturation3/1 -> To Workspace/1, Scope/1, Math Function/1
  Math Function1/1 -> Add to Thrust/2, Add to Yaw/2, Add to Pitch/2, Add to roll/2
  Saturation10/1 -> To Workspace2/1, Scope2/1, Math Function2/1
  ω_2/1 -> Saturation9/1
  ω_4/1 -> Saturation11/1
  C_T/1 -> Product5/3, Product4/1
  Math Function/1 -> Add to Thrust/1, Add to Yaw/1, Add to Pitch/1, Add to roll/1
  Constant/1 -> Product/1
  Constant1/1 -> Product/2
  Product/1 -> Add/2
  Product4/1 -> Add/1
  Product1/1 -> u2/1
  Add to Pitch/1 -> Product2/2
  Product2/1 -> u3/1
  Product3/1 -> Scope5/1, u4/1
  Add/1 -> Scope4/1, u1/1
